simulink model "bbt_lqr_hg_sl"  (Simulink 7.9)
settings: Solver=FixedStepDiscrete  SolverMode=SingleTasking  StartTime=0.0  StopTime=inf  RelTol=1e-3
values from neighbouring files (symbols this model uses):
  F = lqr(Pbb,Q,R)    [bbt_lqr_hg.m]    (also in bbt_lqr_servo_hg.m = Ftmp(:,1:4))
  r1 = 20    [bbt_lqr_hg.m]    (also in bbt_lqr_servo_hg.m = 15; bbt_pid_hg.m = 15)
  ts = 0.02    [sim_param.mat]
undefined symbols (not defined in the file or in its folder): denlpf, numlpf
libraries: arduinolib x4, simulink x3
settings Model: Creator=hirata  LastModifiedBy=hirata  SimulationMode=external  ExtModeTrigDuration=2
settings OptimizationCC: OptimizeModelRefInitCode=on  LifeSpan=1
settings DebuggingCC: SolverPrmCheckMsg=none  StrictBusMsg=Warning
settings HardwareCC: ProdBitPerInt=16  ProdBitPerPointer=8  ProdIntDivRoundTo=Zero  ProdEndianess=LittleEndian  ProdWordSize=8  ProdHWDeviceType=Atmel->AVR
settings RTWCC: SystemTargetFile=realtime.tlc  GenerateMakefile=off  TemplateMakefile=realtime.tmf  Description=Real-Time Toolbox  RTWVerbose=off  ProcessScript=realtime_make_rtw_hook
settings STFCustomTargetCC: TargetLibSuffix=.a  CodeReplacementLibrary=ANSI_C  GenerateSampleERTMain=on  ERTCustomFileBanners=on  SupportNonInlinedSFcns=off  SupportVariableSizeSignals=on  GRTInterface=off  SystemTargetFile=realtime.tlc
settings ERTTargetCC: CodeReplacementLibrary=ANSI_C  MultiwordLength=2048  GenerateSampleERTMain=on  ParMdlRefBuildCompliant=off  CompOptLevelCompliant=off  ConcurrentExecutionCompliant=off  CombineOutputUpdateFcns=off  ERTFirstTimeCompliant=off  SupportContinuousTime=on  SupportVariableSizeSignals=on  ModelStepFunctionPrototypeControlCompliant=off  CPPClassGenCompliant=off  ExtMode=on  ExtModeTransport=3  ExtModeMexFile=ext_serial_win32_comm  ExtModeMexArgs=0 3 115200  InlinedParameterPlacement=NonHierarchical  ERTSrcFileBannerTemplate=realtime_code_template.cgt  ERTHdrFileBannerTemplate=realtime_code_template.cgt  ERTDataSrcFileTemplate=realtime_code_template.cgt  ERTDataHdrFileTemplate=realtime_code_template.cgt  ERTCustomFileTemplate=realtime_file_process.tlc  ConvertIfToSwitch=off  SuppressUnreachableDefaultCases=off
settings SettingsController: Description=Run on Hardware Dialog  TargetExtensionPlatform=Arduino Mega 2560
settings MATStruct: Set_host_COM_port=[0.0]  COM_port_number=1  COM_port_baud_rate=115200  Enable_overrun_detection=[0.0]  Digital_output_to_set_on_overrun=13  Analog_input_reference_voltage=[0.0]  Serial0_baud_rate=9600  Serial1_baud_rate=9600  Serial2_baud_rate=9600  Serial3_baud_rate=9600

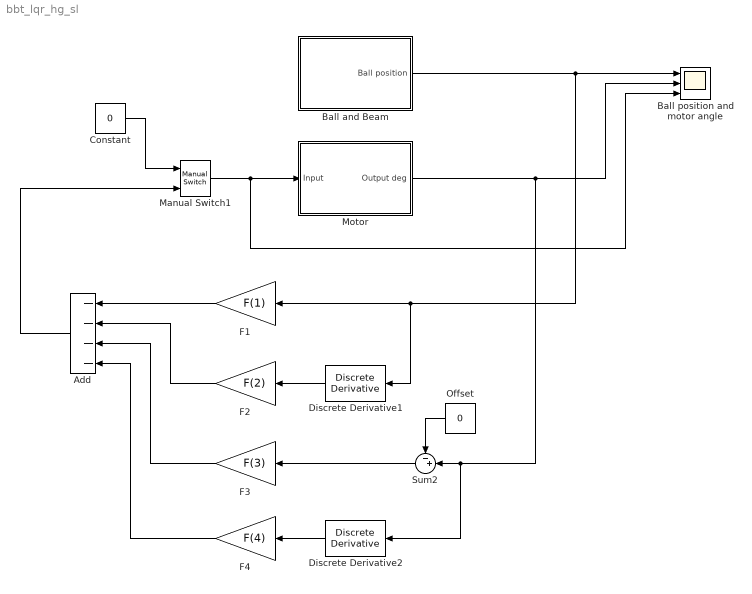
== system bbt_lqr_hg_sl ==
  Add : Sum  Inputs=----
  Ball and Beam : Subsystem
  Ball position and motor angle : Scope  NumInputPorts=3
      settings: TimeRange=30  YMin=-15~-50~-5  YMax=25~50~5
  Constant : Constant  Value=0
  Discrete Derivative1 : simulink/Discrete/Discrete Derivative  gainval=1.0  ICPrevScaledInput=0.0  InputProcessing=Inherited  OutMin=[]  OutMax=[]  OutDataType=fixdt(1, 16)  OutScaling=2^-10  DoSatur=off
  Discrete Derivative2 : simulink/Discrete/Discrete Derivative  gainval=1.0  ICPrevScaledInput=0.0  InputProcessing=Inherited  OutMin=[]  OutMax=[]  OutDataType=fixdt(1, 16)  OutScaling=2^-10  DoSatur=off
  F1 : Gain  Gain=F(1)
  F2 : Gain  Gain=F(2)
  F3 : Gain  Gain=F(3)
  F4 : Gain  Gain=F(4)
  Manual Switch1 : simulink/Signal Routing/Manual Switch  sw=1  action=0  varsize=off
  Motor : Subsystem
  Offset : Constant  Value=0  SampleTime=ts
  Sum2 : Sum  Inputs=-+|
  wires:
  Discrete Derivative1/1 -> F2/1
  Discrete Derivative2/1 -> F4/1
  Ball and Beam/1(Ball position) -> Discrete Derivative1/1, F1/1, Ball position and motor angle/1
  Motor/1(Output deg) -> Sum2/2, Discrete Derivative2/1, Ball position and motor angle/2
  F1/1 -> Add/1
  F2/1 -> Add/2
  F4/1 -> Add/4
  F3/1 -> Add/3
  Add/1 -> Manual Switch1/2
  Sum2/1 -> F3/1
  Offset/1 -> Sum2/1
  Manual Switch1/1 -> Motor/1(Input), Ball position and motor angle/3
  Constant/1 -> Manual Switch1/1

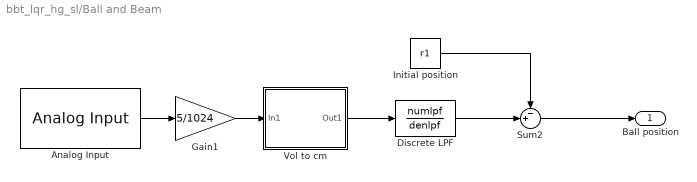
== system bbt_lqr_hg_sl/Ball and Beam ==
  Analog Input : arduinolib/Analog Input  pinNumber=2  sampleTime=ts
  Discrete LPF : DiscreteTransferFcn  Numerator=numlpf  Denominator=denlpf
  Gain1 : Gain  Gain=5/1024
  Initial position : Constant  Value=r1
  Sum2 : Sum  Inputs=-+|
  Vol to cm : Subsystem
  Ball position : Outport
  wires:
  Sum2/1 -> Ball position/1
  Discrete LPF/1 -> Sum2/2
  Initial position/1 -> Sum2/1
  Vol to cm/1(Out1) -> Discrete LPF/1
  Gain1/1 -> Vol to cm/1(In1)
  Analog Input/1 -> Gain1/1

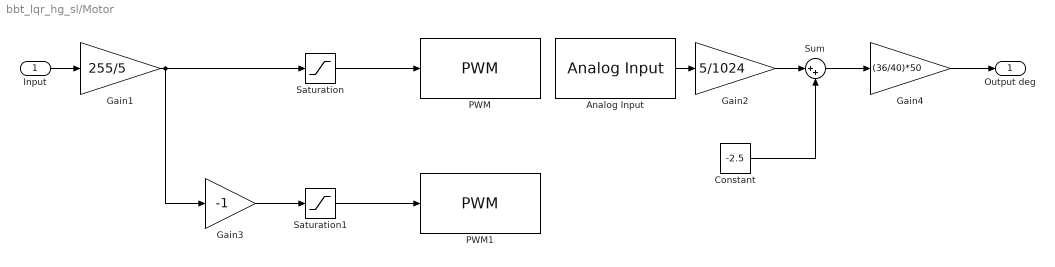
== system bbt_lqr_hg_sl/Motor ==
  Input : Inport
  Analog Input : arduinolib/Analog Input  pinNumber=0  sampleTime=ts
  Constant : Constant  Value=-2.5
  Gain1 : Gain  Gain=255/5
  Gain2 : Gain  Gain=5/1024
  Gain3 : Gain  Gain=-1
  Gain4 : Gain  Gain=(36/40)*50
  PWM : arduinolib/PWM  pinNumber=3
  PWM1 : arduinolib/PWM  pinNumber=5
  Saturation : Saturate  UpperLimit=255  LowerLimit=0
  Saturation1 : Saturate  UpperLimit=255  LowerLimit=0
  Sum : Sum  Inputs=|++
  Output deg : Outport
  wires:
  Gain3/1 -> Saturation1/1
  Constant/1 -> Sum/2
  Sum/1 -> Gain4/1
  Gain2/1 -> Sum/1
  Gain4/1 -> Output deg/1
  Saturation1/1 -> PWM1/1
  Gain1/1 -> Saturation/1, Gain3/1
  Saturation/1 -> PWM/1
  Analog Input/1 -> Gain2/1
  Input/1 -> Gain1/1

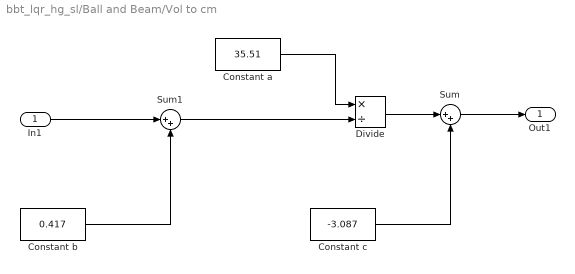
== system bbt_lqr_hg_sl/Ball and Beam/Vol to cm ==
  In1 : Inport
  Constant a : Constant  Value=35.51
  Constant b : Constant  Value=0.417
  Constant c : Constant  Value=-3.087
  Divide : Product  Inputs=*/
  Sum : Sum  Inputs=|++
  Sum1 : Sum  Inputs=|++
  Out1 : Outport
  wires:
  Constant b/1 -> Sum1/2
  Sum1/1 -> Divide/2
  In1/1 -> Sum1/1
  Constant c/1 -> Sum/2
  Sum/1 -> Out1/1
  Divide/1 -> Sum/1
  Constant a/1 -> Divide/1
